simulink model "ShubhamGupta_180749_Lab6_PI"  (R2020b)
settings: Solver=VariableStepAuto  StartTime=0.0  StopTime=250  RelTol=1e-3
settings Model: Creator=sampadasinha  LastModifiedBy=subhamgupta
settings DataIOCC: ReturnWorkspaceOutputs=off

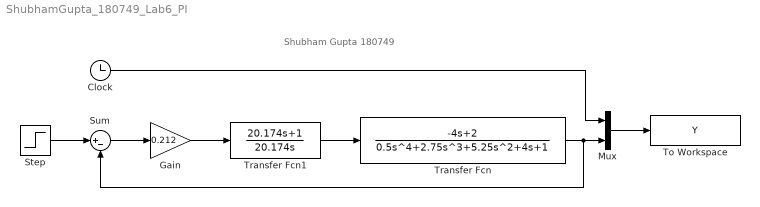
== system ShubhamGupta_180749_Lab6_PI ==
  note: Shubham Gupta 180749
  Clock : Clock
  Gain : Gain  Gain=0.212
  Mux : Mux  Inputs=2
  Step : Step  Time=0  SampleTime=0
  Sum : Sum  Inputs=|+-
  To Workspace : ToWorkspace  VariableName=Y  SampleTime=-1
  Transfer Fcn : TransferFcn  Numerator=[-4 2]  Denominator=[0.5 2.75 5.25 4 1]
  Transfer Fcn1 : TransferFcn  Numerator=[20.174 1]  Denominator=[20.174 0]
  wires:
  Sum/1 -> Gain/1
  Clock/1 -> Mux/1
  Mux/1 -> To Workspace/1
  Step/1 -> Sum/1
  Transfer Fcn/1 -> Sum/2, Mux/2
  Gain/1 -> Transfer Fcn1/1
  Transfer Fcn1/1 -> Transfer Fcn/1
